simulink model "PID_Difuso"  (R2015a)
settings: Solver=ode4  StartTime=0.0  StopTime=100.0  RelTol=1e-3
undefined symbols (not defined in the file): g, k, l, m
libraries: fuzblock x1
settings Model: Creator=Benjamin Nicolas  LastModifiedBy=Benjamin Nicolas

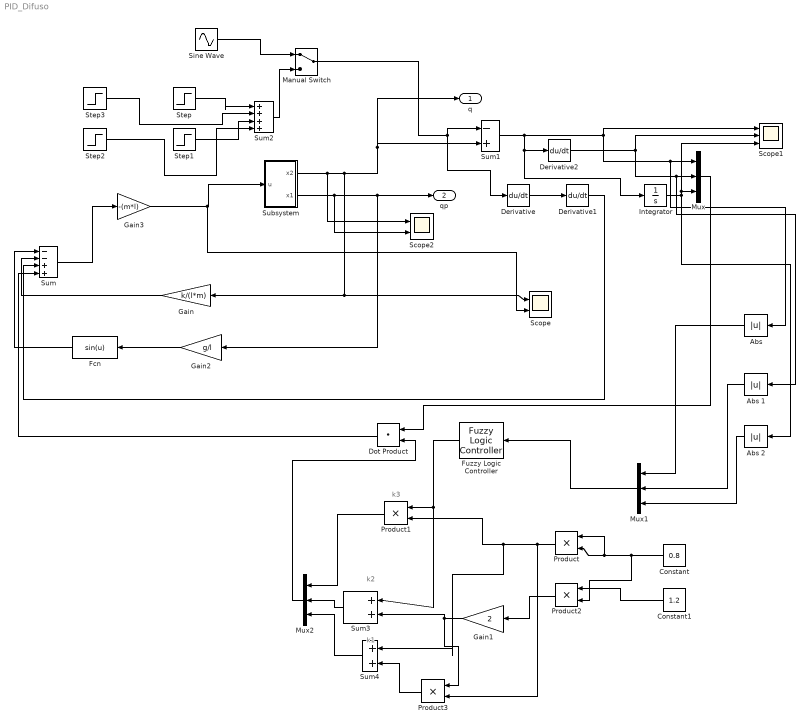
== system PID_Difuso ==
  note: k1
  note: k2
  note: k3
  "Abs\t" : Abs
  Abs	1 : Abs
  Abs	2 : Abs
  Constant : Constant  Value=0.8
  Constant1 : Constant  Value=1.2
  Derivative : Derivative
  Derivative1 : Derivative
  Derivative2 : Derivative
  Dot Product : DotProduct  InputSameDT=on  OutDataTypeStr=Inherit: Inherit via internal rule
  Fcn : Fcn  Expr=sin(u)
  Fuzzy Logic Controller : fuzblock/Fuzzy Logic  Controller  fis=P_Difuso
  Gain : Gain  Gain=k/(l*m)
  Gain1 : Gain  Gain=2
  Gain2 : Gain  Gain=g/l
  Gain3 : Gain  Gain=-(m*l)
  Integrator : Integrator
  Manual Switch : ManualSwitch
  Mux : Mux  Inputs=3
  Mux1 : Mux  Inputs=3
  Mux2 : Mux  Inputs=3
  Product{,1..3} (4 alike) : Product
  Scope : Scope  NumInputPorts=2
      settings: YMin=-5~-5  YMax=5~5
  Scope1 : Scope  NumInputPorts=3
      settings: YMin=-5~-5~-5  YMax=5~5~5
  Scope2 : Scope  NumInputPorts=2
      settings: YMin=-5~-5  YMax=5~5  SaveName=ScopeData2
  Sine Wave : Sin  SampleTime=0
  Step : Step  Time=10  After=10  SampleTime=0
  Step1 : Step  Time=10  Before=-20  After=-15  SampleTime=0
  Step2 : Step  Time=10  Before=-15  After=20  SampleTime=0
  Step3 : Step  Time=10  Before=10  After=-20  SampleTime=0
  Subsystem : Subsystem
  Sum : Sum  Inputs=|--++
  Sum1 : Sum  Inputs=|-+
  Sum2 : Sum  Inputs=|++++
  Sum3 : Sum  Inputs=|++
  Sum4 : Sum  Inputs=|++
  "q " : Outport
  "qp " : Outport  Port=2
  wires:
  Subsystem/1("x2 ") -> Scope2/1, Scope/1, Gain/1, Sum1/2, "q "/1
  Subsystem/2("x1 ") -> Scope2/2, Gain2/1, "qp "/1
  Manual Switch/1 -> Derivative/1, Sum1/1
  Gain3/1 -> Subsystem/1("u "), Scope/2
  Sum/1 -> Gain3/1
  Gain/1 -> Sum/2
  Derivative/1 -> Derivative1/1
  Sum1/1 -> "Abs\t"/1, Mux/1, Scope1/1, Integrator/1, Derivative2/1
  Derivative2/1 -> Abs	1/1, Mux/2, Scope1/2
  Fcn/1 -> Sum/1
  Gain2/1 -> Fcn/1
  Derivative1/1 -> Sum/3
  Mux/1 -> Dot Product/1
  Integrator/1 -> Scope1/3, Mux/3, Abs	2/1
  Sum2/1 -> Manual Switch/2
  Step/1 -> Sum2/1
  Step3/1 -> Sum2/2
  Step1/1 -> Sum2/3
  Step2/1 -> Sum2/4
  Sine Wave/1 -> Manual Switch/1
  Dot Product/1 -> Sum/4
  "Abs\t"/1 -> Mux1/1
  Abs	1/1 -> Mux1/2
  Abs	2/1 -> Mux1/3
  Mux1/1 -> Fuzzy Logic Controller/1
  Constant/1 -> Product2/2, Product/1, Product/2
  Fuzzy Logic Controller/1 -> Sum3/1, Product1/1
  Constant1/1 -> Product2/1
  Product2/1 -> Gain1/1
  Gain1/1 -> Product3/1, Sum3/2
  Product/1 -> Product3/2, Sum4/1, Product1/2
  Product3/1 -> Sum4/2
  Sum4/1 -> Mux2/3
  Sum3/1 -> Mux2/2
  Product1/1 -> Mux2/1
  Mux2/1 -> Dot Product/2

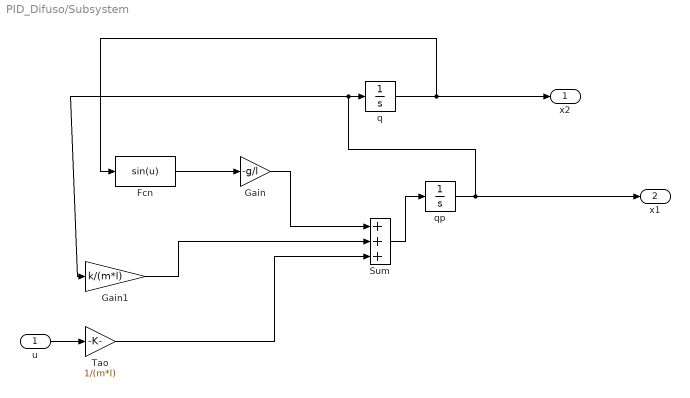
== system PID_Difuso/Subsystem ==
  "u " : Inport
  Fcn : Fcn  Expr=sin(u)
  Gain : Gain  Gain=-g/l
  Gain1 : Gain  Gain=k/(m*l)
  Sum : Sum  Inputs=+++
  "Tao " : Gain  Gain=1/(m*l)
  q : Integrator
  qp : Integrator
  "x2 " : Outport
  "x1 " : Outport  Port=2
  wires:
  Sum/1 -> qp/1
  "u "/1 -> "Tao "/1
  Gain1/1 -> Sum/2
  Gain/1 -> Sum/1
  q/1 -> "x2 "/1, Fcn/1
  Fcn/1 -> Gain/1
  qp/1 -> "x1 "/1, q/1, Gain1/1
  "Tao "/1 -> Sum/3
